simulink model "MCUSoftware"  (R2017b)
settings: Solver=FixedStepAuto  StartTime=0.0  StopTime=inf  RelTol=1e-3
undefined symbols (not defined in the file): Down, GPTRIP1SEL, GPTRIP2SEL, TZ1, TZ2, Up
libraries: c2802xlib x7, c2807xlib x2, c280xlib x1
settings Model: ExtModeTrigDuration=8  Creator=Joergen  LastModifiedBy=Joergen
settings OptimizationCC: DefaultUnderspecifiedDataType=single  PassReuseOutputArgsAs=Individual arguments  MaxStackSize=512
settings DebuggingCC: ParameterTunabilityLossMsg=error
settings HardwareCC: ProdBitPerChar=16  ProdBitPerInt=16  ProdBitPerPointer=32  ProdBitPerSizeT=32  ProdBitPerPtrDiffT=32  ProdLargestAtomicInteger=Integer  ProdLargestAtomicFloat=None  ProdWordSize=16  ProdLongLongMode=on  ProdHWDeviceType=Texas Instruments->C2000
settings SFSimCC: MATLABDynamicMemAlloc=off
settings RTWCC: SystemTargetFile=ert.tlc  HardwareBoard=TI Piccolo F2807x  TLCOptions=-aInlineSetEventsForThisBaseRateFcn=TLC_FALSE -aSuppressMultiTaskScheduler=TLC_FALSE -aRateBasedStepFcn=1  TemplateMakefile=ert_default_tmf  GenerateReport=on  Toolchain=Texas Instruments Code Composer Studio (C2000)  BuildConfiguration=Specify  IncludeHyperlinkInReport=on  LaunchReport=on  GenerateTraceInfo=on  GenerateTraceReport=on  GenerateTraceReportSl=on  GenerateTraceReportSf=on  GenerateTraceReportEml=on
settings CodeAppCC: ForceParamTrailComments=on  IgnoreCustomStorageClasses=off  OperatorAnnotations=on  SimulinkDataObjDesc=on  SFDataObjDesc=on  InsertBlockDesc=on
settings ERTTargetCC: CodeReplacementLibrary=TI C28x  SupportContinuousTime=on

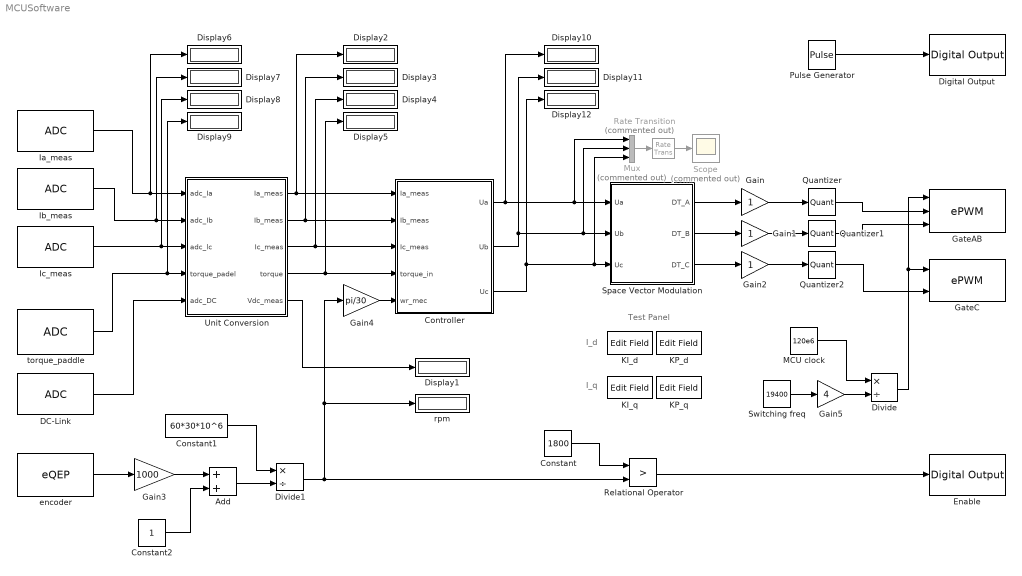
== system MCUSoftware ==
  note: I_d
  note: I_q
  note: Test Panel
  Add : Sum
  Constant : Constant  Value=1800
  Constant1 : Constant  Value=60*30*10^6
  Constant2 : Constant
  "Controller " : Subsystem
  DC-Link : c2802xlib/ADC  ADCModule=D  samplingMode=Single sample mode  ADCResolution=12-bit (Single-ended input)  useSOC1=SOC1  useSOC2=SOC0_SOC1  SOCAcquisitionWindow=12  SOCTriggerSource=ePWM1_ADCSOCA  SOCInterruptTrigger=No ADCINT  Ts=0.00001  dType=uint16  postInterrupt=off  interruptSel=ADCINT1  ADCINTContinuous=on  endma=off  chdma=1  blkParamProc=C2000_Type4  conv1=ADCINA0  conv2=ADCINA0 and ADCINB0  conv1_Type4=ADCIN1  conv2_Type4=ADCIN0 and ADCIN1
      settings: SourceProductName=Embedded Coder Support Package for Texas Instruments C2000 Processors
  Digital Output : c2807xlib/Digital Output  GPIO_Number=GPIO24~GPIO31  GPIO_Bit0=off  GPIO_BIT0_Toggle=off  GPIO_Bit1=off  GPIO_BIT1_Toggle=off  GPIO_Bit2=off  GPIO_BIT2_Toggle=off  GPIO_Bit3=off  GPIO_BIT3_Toggle=off  GPIO_Bit4=off  GPIO_BIT4_Toggle=off  GPIO_Bit5=off  GPIO_BIT5_Toggle=off  GPIO_Bit6=off  GPIO_BIT6_Toggle=on  GPIO_Bit7=on  GPIO_BIT7_Toggle=off
      settings: SourceProductName=Embedded Coder Support Package for Texas Instruments C2000 Processors  SourceProductBaseCode=TIC2000
  Display{1..12} (12 alike) : Display
  Divide : Product  Inputs=*/
  Divide1 : Product  Inputs=*/
  Enable : c2807xlib/Digital Output  GPIO_Number=GPIO8~GPIO15  GPIO_Bit0=off  GPIO_BIT0_Toggle=off  GPIO_Bit1=off  GPIO_BIT1_Toggle=off  GPIO_Bit2=off  GPIO_BIT2_Toggle=off  GPIO_Bit3=off  GPIO_BIT3_Toggle=off  GPIO_Bit4=off  GPIO_BIT4_Toggle=off  GPIO_Bit5=on  GPIO_BIT5_Toggle=off  GPIO_Bit6=off  GPIO_BIT6_Toggle=on  GPIO_Bit7=off  GPIO_BIT7_Toggle=off
      settings: SourceProductName=Embedded Coder Support Package for Texas Instruments C2000 Processors  SourceProductBaseCode=TIC2000
  Gain : Gain
  Gain1 : Gain
  Gain2 : Gain
  Gain3 : Gain  Gain=1000
  Gain4 : Gain  Gain=pi/30
  Gain5 : Gain  Gain=4
  "GateAB " : c2802xlib/ePWM  useModule=ePWM1  ePWMxLINKTBPRD=Not Linked  periodUnits=Clock cycles  timerSource=Input port  timerPeriod_clk=64000  timerPeriod_sec=0.0001  tbshadow=Counter equals to zero  countingMode=Up-Down  phaseActiveEnable=Disable  phaseDirection=Count down after sync  phaseActive=0  synchronizationEnable=off  dcaevt1Sync=off  dcbevt1Sync=off  synchronizationOption=Disable  clockPrescale=1  HSclockPrescale=1  enswap=off  ePWMxAStatus=on  ePWMxAactionLogic1=Set  ePWMxAactionLogic2=Clear  ePWMxAactionLogic3=Clear  ePWMxAactionLogic4=Set  ePWMxAactionLogic5=Do nothing  ePWMxAactionLogic6=Do nothing  ePWMxALoadMode=Load on counter equals to zero (CTR=Zero)  ePWMxACSFenable=off  ePWMxACSFvalue=Forcing disable  ePWMxASFreload=Zero  ePWMxBStatus=on  ePWMxBactionLogic1=Set  ePWMxBactionLogic2=Clear  ePWMxBactionLogic3=Do nothing  ePWMxBactionLogic4=Do nothing  ePWMxBactionLogic5=Clear  ePWMxBactionLogic6=Set  ePWMxBLoadMode=Load on counter equals to zero (CTR=Zero)  ePWMxBCSFenable=off  ePWMxBCSFvalue=Forcing disable  ePWMxBSFreload=Zero  ePWNxBOutWay=off  ePWMxLINKCMPA=Not Linked  CMPAUnits=Percentages  CMPASource=Input port  CMPAValue_per=50  CMPAValue_clk=0  enCMPAshadow=Counter equals to zero  ePWMxLINKCMPB=Not Linked  CMPBUnits=Percentages  CMPBSource=Input port  CMPBValue_per=50  CMPBValue_clk=0  enCMPBshadow=Counter equals to zero  ePWMxLINKCMPC=Not Linked  CMPCUnits=Clock cycles  CMPCSource=Specify via dialog  CMPCValue_per=50  CMPCValue_clk=32000  enCMPCshadow=Counter equals to zero  ePWMxLINKCMPD=Not Linked  CMPDUnits=Clock cycles  CMPDSource=Specify via dialog  CMPDValue_per=50  CMPDValue_clk=32000  enCMPDshadow=Counter equals to zero  enableDBePWMxA=off  enableDBePWMxB=off  enhalfcycle=off  DBpolarity=Active high (AH)  DBedgeDelay=Positive  DBSource_ePWMxA=ePWMxA  DBSource_ePWMxB=ePWMxA  DBperiodSource=Specify via dialog  REDperiod=0  FEDperiod=0  adcstartModuleA=on  adcrequestEventA=First event  adcstartEventA=Digital Compare Module A Event 1 start of conversion (DCAEVT1.soc)  adcstartEventA_type2=Counter equals to period (CTR=PRD)  adcstartModuleB=off  adcrequestEventB=First event  adcstartEventB=Counter equals to zero (CTR=Zero)  adcstartEventB_type2=Counter equals to zero (CTR=Zero)  intEn=off  intPrd=First event  intSel=Counter equals to zero (CTR=Zero)  intSel_type2=Counter equals to zero (CTR=Zero)  hrpe=off  enHRPWM=off  HRPWM_LoadMode=Counter equals to period (CTR=PRD)  HRPWM_CTLMode=Duty or Period control mode  HRPWM_EDGMode=Both edge  hrpeb=off  enHRPWMB=off  HRPWM_LoadModeB=Counter equals to zero (CTR=ZERO)  HRPWM_CTLModeB=Duty or Period control mode  HRPWM_EDGModeB=Both edge  enSFO=on  enautoconv=on  chopperEnable=off  chopperFrequency=1  chopperFirstwidth=1  chopperDuty=12.5%  tripZonesource=Specify via dialog  tzselOSHT1=off  tzselOSHT2=off  tzselOSHT3=off  tzselOSHDCAEV1=off  tzselOSHDCBEV1=off  tzselCBC1=off  tzselCBC2=off  tzselCBC3=off  tzselCBCDCAEV2=off  tzselCBCDCBEV2=off  tzselOSHT4=off  tzselOSHT5=off  tzselOSHT6=off  tzselCBC4=off  tzselCBC5=off  tzselCBC6=off  enTzOstIntr=off  enTzCbcIntr=off  enTzDCAEVT1Intr=off  enTzDCAEVT2Intr=off  enTzDCBEVT1Intr=off  enTzDCBEVT2Intr=off  ePWMxAforced=No action  ePWMxBforced=No action  DCAEVT1forced=No action  DCBEVT1forced=No action  DCAEVT2forced=No action  DCBEVT2forced=No action  dcah=Trip Zone 1 input (TZ1)  dcal=Trip Zone 2 input (TZ2)  dcbh=Trip Zone 1 input (TZ1)  dcbl=Trip Zone 2 input (TZ2)  dcah_type2=GPTRIP1SEL/(TZ1)  dcal_type2=GPTRIP2SEL/(TZ2)  dcbh_type2=GPTRIP1SEL/(TZ1)  dcbl_type2=GPTRIP2SEL/(TZ2)  gendcaevt1=Event disabled  gendcaevt2=Event disabled  gendcbevt1=Event disabled  gendcbevt2=Event disabled  dcaevt1src=DCAEVT1 with sync  dcaevt2src=DCAEVT2 with sync  dcbevt1src=DCBEVT1 with sync  dcbevt2src=DCBEVT2 with sync  pulsesel=Counter equals to zero (CTR=Zero)  blankinv=off  blankoffset=0  blankwidth=0  evsrcsel=Filtered version of DCAEVT1 (DCAEVT1FILT)  encape=off  PwmType=C2000_Type4
      settings: SourceProductName=Embedded Coder Support Package for Texas Instruments C2000 Processors
  GateC : c2802xlib/ePWM  useModule=ePWM2  ePWMxLINKTBPRD=Not Linked  periodUnits=Clock cycles  timerSource=Input port  timerPeriod_clk=64000  timerPeriod_sec=0.0001  tbshadow=Counter equals to zero  countingMode=Up-Down  phaseActiveEnable=Disable  phaseDirection=Count down after sync  phaseActive=0  synchronizationEnable=off  dcaevt1Sync=off  dcbevt1Sync=off  synchronizationOption=Disable  clockPrescale=1  HSclockPrescale=1  enswap=off  ePWMxAStatus=on  ePWMxAactionLogic1=Set  ePWMxAactionLogic2=Clear  ePWMxAactionLogic3=Clear  ePWMxAactionLogic4=Set  ePWMxAactionLogic5=Do nothing  ePWMxAactionLogic6=Do nothing  ePWMxALoadMode=Load on counter equals to zero (CTR=Zero)  ePWMxACSFenable=off  ePWMxACSFvalue=Forcing disable  ePWMxASFreload=Zero  ePWMxBStatus=off  ePWMxBactionLogic1=Set  ePWMxBactionLogic2=Clear  ePWMxBactionLogic3=Do nothing  ePWMxBactionLogic4=Do nothing  ePWMxBactionLogic5=Clear  ePWMxBactionLogic6=Set  ePWMxBLoadMode=Load on counter equals to zero (CTR=Zero)  ePWMxBCSFenable=off  ePWMxBCSFvalue=Forcing disable  ePWMxBSFreload=Zero  ePWNxBOutWay=off  ePWMxLINKCMPA=Not Linked  CMPAUnits=Percentages  CMPASource=Input port  CMPAValue_per=50  CMPAValue_clk=0  enCMPAshadow=Counter equals to zero  ePWMxLINKCMPB=Not Linked  CMPBUnits=Clock cycles  CMPBSource=Specify via dialog  CMPBValue_per=50  CMPBValue_clk=32000  enCMPBshadow=Counter equals to zero  ePWMxLINKCMPC=Not Linked  CMPCUnits=Clock cycles  CMPCSource=Specify via dialog  CMPCValue_per=50  CMPCValue_clk=32000  enCMPCshadow=Counter equals to zero  ePWMxLINKCMPD=Not Linked  CMPDUnits=Clock cycles  CMPDSource=Specify via dialog  CMPDValue_per=50  CMPDValue_clk=32000  enCMPDshadow=Counter equals to zero  enableDBePWMxA=off  enableDBePWMxB=off  enhalfcycle=off  DBpolarity=Active high (AH)  DBedgeDelay=Positive  DBSource_ePWMxA=ePWMxA  DBSource_ePWMxB=ePWMxA  DBperiodSource=Specify via dialog  REDperiod=0  FEDperiod=0  adcstartModuleA=off  adcrequestEventA=First event  adcstartEventA=Digital Compare Module A Event 1 start of conversion (DCAEVT1.soc)  adcstartEventA_type2=Digital Compare Module A Event 1 start of conversion (DCAEVT1.soc)  adcstartModuleB=off  adcrequestEventB=First event  adcstartEventB=Counter equals to zero (CTR=Zero)  adcstartEventB_type2=Counter equals to zero (CTR=Zero)  intEn=off  intPrd=First event  intSel=Counter equals to zero (CTR=Zero)  intSel_type2=Counter equals to zero (CTR=Zero)  hrpe=off  enHRPWM=off  HRPWM_LoadMode=Counter equals to period (CTR=PRD)  HRPWM_CTLMode=Duty or Period control mode  HRPWM_EDGMode=Both edge  hrpeb=off  enHRPWMB=off  HRPWM_LoadModeB=Counter equals to zero (CTR=ZERO)  HRPWM_CTLModeB=Duty or Period control mode  HRPWM_EDGModeB=Both edge  enSFO=on  enautoconv=on  chopperEnable=off  chopperFrequency=1  chopperFirstwidth=1  chopperDuty=12.5%  tripZonesource=Specify via dialog  tzselOSHT1=off  tzselOSHT2=off  tzselOSHT3=off  tzselOSHDCAEV1=off  tzselOSHDCBEV1=off  tzselCBC1=off  tzselCBC2=off  tzselCBC3=off  tzselCBCDCAEV2=off  tzselCBCDCBEV2=off  tzselOSHT4=off  tzselOSHT5=off  tzselOSHT6=off  tzselCBC4=off  tzselCBC5=off  tzselCBC6=off  enTzOstIntr=off  enTzCbcIntr=off  enTzDCAEVT1Intr=off  enTzDCAEVT2Intr=off  enTzDCBEVT1Intr=off  enTzDCBEVT2Intr=off  ePWMxAforced=No action  ePWMxBforced=No action  DCAEVT1forced=No action  DCBEVT1forced=No action  DCAEVT2forced=No action  DCBEVT2forced=No action  dcah=Trip Zone 1 input (TZ1)  dcal=Trip Zone 2 input (TZ2)  dcbh=Trip Zone 1 input (TZ1)  dcbl=Trip Zone 2 input (TZ2)  dcah_type2=GPTRIP1SEL/(TZ1)  dcal_type2=GPTRIP2SEL/(TZ2)  dcbh_type2=GPTRIP1SEL/(TZ1)  dcbl_type2=GPTRIP2SEL/(TZ2)  gendcaevt1=Event disabled  gendcaevt2=Event disabled  gendcbevt1=Event disabled  gendcbevt2=Event disabled  dcaevt1src=DCAEVT1 with sync  dcaevt2src=DCAEVT2 with sync  dcbevt1src=DCBEVT1 with sync  dcbevt2src=DCBEVT2 with sync  pulsesel=Counter equals to zero (CTR=Zero)  blankinv=off  blankoffset=0  blankwidth=0  evsrcsel=Filtered version of DCAEVT1 (DCAEVT1FILT)  encape=off  PwmType=C2000_Type4
      settings: SourceProductName=Embedded Coder Support Package for Texas Instruments C2000 Processors
  Ia_meas : c2802xlib/ADC  ADCModule=A  samplingMode=Single sample mode  ADCResolution=12-bit (Single-ended input)  useSOC1=SOC0  useSOC2=SOC0_SOC1  SOCAcquisitionWindow=12  SOCTriggerSource=ePWM1_ADCSOCA  SOCInterruptTrigger=No ADCINT  Ts=0.00001  dType=uint16  postInterrupt=off  interruptSel=ADCINT1  ADCINTContinuous=on  endma=off  chdma=1  blkParamProc=C2000_Type4  conv1=ADCINA0  conv2=ADCINA0 and ADCINB0  conv1_Type4=ADCIN0  conv2_Type4=ADCIN0 and ADCIN1
      settings: SourceProductName=Embedded Coder Support Package for Texas Instruments C2000 Processors
  "Ib_meas " : c2802xlib/ADC  ADCModule=B  samplingMode=Single sample mode  ADCResolution=12-bit (Single-ended input)  useSOC1=SOC0  useSOC2=SOC0_SOC1  SOCAcquisitionWindow=12  SOCTriggerSource=ePWM1_ADCSOCA  SOCInterruptTrigger=ADCINT1  Ts=0.00001  dType=uint16  postInterrupt=off  interruptSel=ADCINT1  ADCINTContinuous=on  endma=off  chdma=1  blkParamProc=C2000_Type4  conv1=ADCINA0  conv2=ADCINA0 and ADCINB0  conv1_Type4=ADCIN0  conv2_Type4=ADCIN0 and ADCIN1
      settings: SourceProductName=Embedded Coder Support Package for Texas Instruments C2000 Processors
  "Ic_meas " : c2802xlib/ADC  ADCModule=D  samplingMode=Single sample mode  ADCResolution=12-bit (Single-ended input)  useSOC1=SOC0  useSOC2=SOC0_SOC1  SOCAcquisitionWindow=12  SOCTriggerSource=ePWM1_ADCSOCA  SOCInterruptTrigger=ADCINT1  Ts=0.00001  dType=uint16  postInterrupt=off  interruptSel=ADCINT1  ADCINTContinuous=on  endma=off  chdma=1  blkParamProc=C2000_Type4  conv1=ADCINA0  conv2=ADCINA0 and ADCINB0  conv1_Type4=ADCIN0  conv2_Type4=ADCIN0 and ADCIN1
      settings: SourceProductName=Embedded Coder Support Package for Texas Instruments C2000 Processors
  KI_d : EditField  WebBlockId=101  ModelName=MCUSoftware  LabelPosition=Hide  ShowInitialText=off  Alignment=Center
  KI_q : EditField  WebBlockId=102  ModelName=MCUSoftware  LabelPosition=Hide  ShowInitialText=off  Alignment=Center
  KP_d : EditField  WebBlockId=103  ModelName=MCUSoftware  LabelPosition=Hide  ShowInitialText=off  Alignment=Center
  KP_q : EditField  WebBlockId=104  ModelName=MCUSoftware  LabelPosition=Hide  ShowInitialText=off  Alignment=Center
  MCU clock : Constant  Value=120e6
  Mux : Mux  Commented=on  Inputs=3
  Pulse Generator : DiscretePulseGenerator  PulseType=Time based  Period=0.5  PulseWidth=90
  Quantizer : Quantizer  QuantizationInterval=0.001
  Quantizer1 : Quantizer  QuantizationInterval=0.001
  Quantizer2 : Quantizer  QuantizationInterval=0.001
  Rate Transition : RateTransition  Commented=on
  Relational Operator : RelationalOperator  Operator=>  RndMeth=Simplest
  Scope : Scope  Commented=on
  Space Vector Modulation : Subsystem
  Switching freq : Constant  Value=19400
  Unit Conversion : Subsystem
  encoder : c280xlib/eQEP  useModule=eQEP1  pcInputmode=Quadrature-count  externalClockrate=2x resolution: Count the rising/falling edge  swapPolarityselection=Clockwise  qdfOutputport=off  qapPolarityselection=off  qbpPolarityselection=off  qipPolarityselection=off  qspPolarityselection=off  igatePolarityselection=off  sampleTime=0.00001  pcOutputport=off  pcMaximumvalue=4294967295  indexInitializationcheck=off  indexInitializationevent=Rising edge  strobeInitializationcheck=off  strobeInitializationevent=Rising edge  softwareInitializationcheck=off  softwareInitializationsource=Set to init value at start up  softwareInitializationmode=on  pcInitialvalue=2147483648  pcResetmode=Reset on an index event  ieloutputport=off  indexEventlatch=Rising edge  seloutputport=off  strobeEventlatch=Rising edge  pcefOutputport=off  enableEqepcapture=on  qctmrOutputport=off  qcprdOutputport=on  captureTimerprescaler=128  upEventprescaler=128  overflowErrorflag=off  directionErrorflag=off  captureTimerposition=On position counter read  unitTimerperiod=100000000  captureTimerlatch=off  capturePeriodlatch=off  positionCounterlatch=off  soenPolarityselection=off  spselPolarityselection=Index pin is used for sync output  compareValuesource=Specify via dialog  shadowMode=Load on QPOSCNT=0  compareValue=4294967295  syncOutputwidth=1  polaritySyncoutput=Active high  watchdogEnable=off  watchdogTimer=65535  outport1Datatype=auto  outport2Datatype=auto  outport3Datatype=auto  outport4Datatype=auto  outport5Datatype=auto  outport6Datatype=auto  outport7Datatype=auto  outport8Datatype=auto  outport9Datatype=auto  outport10Datatype=auto  outport11Datatype=auto  outport12Datatype=auto  eqepinterrupt_pce=off  eqepinterrupt_qpe=off  eqepinterrupt_qdc=off  eqepinterrupt_wto=off  eqepinterrupt_pcu=off  eqepinterrupt_pco=off  eqepinterrupt_pcr=off  eqepinterrupt_pcm=off  eqepinterrupt_sel=off  eqepinterrupt_iel=off  eqepinterrupt_uto=off  pheOutputport=off  watchdogOutputport=off  outport13Datatype=auto  outport14Datatype=auto
      settings: SourceProductName=Embedded Coder Support Package for Texas Instruments C2000 Processors  SourceProductBaseCode=TIC2000
  rpm : Display
  torque_paddle : c2802xlib/ADC  ADCModule=B  samplingMode=Single sample mode  ADCResolution=12-bit (Single-ended input)  useSOC1=SOC1  useSOC2=SOC0_SOC1  SOCAcquisitionWindow=12  SOCTriggerSource=ePWM1_ADCSOCA  SOCInterruptTrigger=No ADCINT  Ts=0.00001  dType=uint16  postInterrupt=off  interruptSel=ADCINT1  ADCINTContinuous=on  endma=off  chdma=1  blkParamProc=C2000_Type4  conv1=ADCINA0  conv2=ADCINA0 and ADCINB0  conv1_Type4=ADCIN1  conv2_Type4=ADCIN0 and ADCIN1
      settings: SourceProductName=Embedded Coder Support Package for Texas Instruments C2000 Processors
  wires:
  torque_paddle/1 -> Unit Conversion/4(torque_padel), Display9/1
  Unit Conversion/3(Ic_meas) -> Display4/1, "Controller "/3(Ic_meas)
  "Ic_meas "/1 -> Unit Conversion/3(adc_lc), Display8/1
  Unit Conversion/2(Ib_meas) -> Display3/1, "Controller "/2(Ib_meas)
  "Ib_meas "/1 -> Unit Conversion/2(adc_Ib), Display7/1
  Relational Operator/1 -> Enable/1
  Gain2/1 -> Quantizer2/1
  Divide/1 -> "GateAB "/1, GateC/1
  Gain1/1 -> Quantizer1/1
  "Controller "/3(Uc) -> Space Vector Modulation/3(Uc), Mux/3, Display12/1
  Unit Conversion/4(torque) -> Display5/1, "Controller "/4(torque_in)
  Mux/1 -> Rate Transition/1
  Space Vector Modulation/3(DT_C) -> Gain2/1
  Space Vector Modulation/1(DT_A) -> Gain/1
  "Controller "/2(Ub) -> Mux/2, Space Vector Modulation/2(Ub), Display11/1
  Space Vector Modulation/2(DT_B) -> Gain1/1
  Ia_meas/1 -> Display6/1, Unit Conversion/1(adc_Ia)
  Gain/1 -> Quantizer/1
  DC-Link/1 -> Unit Conversion/5(adc_DC)
  Unit Conversion/5(Vdc_meas) -> Display1/1
  Quantizer/1 -> "GateAB "/2
  Quantizer1/1 -> "GateAB "/3
  Quantizer2/1 -> GateC/2
  Pulse Generator/1 -> Digital Output/1
  Unit Conversion/1(Ia_meas) -> "Controller "/1(Ia_meas), Display2/1
  MCU clock/1 -> Divide/1
  Switching freq/1 -> Gain5/1
  Rate Transition/1 -> Scope/1
  "Controller "/1(Ua) -> Space Vector Modulation/1(Ua), Mux/1, Display10/1
  Divide1/1 -> Relational Operator/2, Gain4/1, rpm/1
  Gain3/1 -> Add/1
  Constant1/1 -> Divide1/1
  Gain4/1 -> "Controller "/5(wr_mec)
  Gain5/1 -> Divide/2
  Constant/1 -> Relational Operator/1
  Add/1 -> Divide1/2
  encoder/1 -> Gain3/1
  Constant2/1 -> Add/2

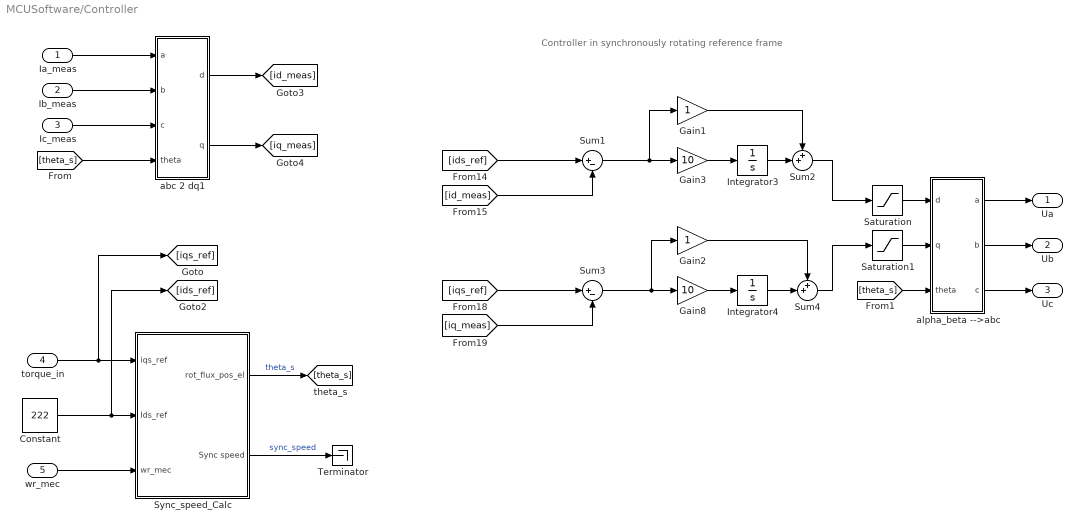
== system MCUSoftware/Controller  ==
  note: Controller in synchronously rotating reference frame
  Ia_meas : Inport
  Ib_meas : Inport  Port=2
  Ic_meas : Inport  Port=3
  torque_in : Inport  Port=4
  wr_mec : Inport  Port=5
  " alpha_beta -->abc" : Subsystem
  Constant : Constant  Value=222
  Gain1 : Gain  SaturateOnIntegerOverflow=on  OutDataTypeStr=Inherit: Same as input  ParamDataTypeStr=Inherit: Same as input
  Gain2 : Gain  SaturateOnIntegerOverflow=on  OutDataTypeStr=Inherit: Same as input  ParamDataTypeStr=Inherit: Same as input
  Gain3 : Gain  Gain=10  SaturateOnIntegerOverflow=on  OutDataTypeStr=Inherit: Same as input  ParamDataTypeStr=Inherit: Same as input
  Gain8 : Gain  Gain=10  SaturateOnIntegerOverflow=on  OutDataTypeStr=Inherit: Same as input  ParamDataTypeStr=Inherit: Same as input
  Integrator3 : Integrator
  Integrator4 : Integrator
  Saturation : Saturate  UpperLimit=34  LowerLimit=-34
  Saturation1 : Saturate  UpperLimit=34  LowerLimit=-34
  Sum1 : Sum  Inputs=|+-  SaturateOnIntegerOverflow=on  InputSameDT=on  OutDataTypeStr=Inherit: Same as first input
  Sum2 : Sum  Inputs=++|  SaturateOnIntegerOverflow=on  InputSameDT=on  OutDataTypeStr=Inherit: Same as first input
  Sum3 : Sum  Inputs=|+-  SaturateOnIntegerOverflow=on  InputSameDT=on  OutDataTypeStr=Inherit: Same as first input
  Sum4 : Sum  Inputs=++|  SaturateOnIntegerOverflow=on  InputSameDT=on  OutDataTypeStr=Inherit: Same as first input
  Sync_speed_Calc : Subsystem
  Terminator : Terminator
  abc 2 dq1 : Subsystem
  Ua : Outport
  Ub : Outport  Port=2
  Uc : Outport  Port=3
  wires:
  Ia_meas/1 -> abc 2 dq1/1(a)
  Ic_meas/1 -> abc 2 dq1/3(c)
  torque_in/1 -> [iqs_ref], Sync_speed_Calc/1(iqs_ref)
  Constant/1 -> [ids_ref], Sync_speed_Calc/2(Ids_ref)
  wr_mec/1 -> Sync_speed_Calc/3(wr_mec)
  Sync_speed_Calc/1(rot_flux_pos_el) -> [theta_s]  "theta_s"
  [theta_s] -> abc 2 dq1/4(theta)
  Integrator4/1 -> Sum4/2
  Integrator3/1 -> Sum2/2
  [iq_meas] -> Sum3/2
  [iqs_ref] -> Sum3/1
  Gain8/1 -> Integrator4/1
  Gain3/1 -> Integrator3/1
  Sum4/1 -> Saturation1/1
  abc 2 dq1/1(d) -> [id_meas]
  abc 2 dq1/2(q) -> [iq_meas]
  [theta_s] -> " alpha_beta -->abc"/3(theta)
  Sum2/1 -> Saturation/1
  Ib_meas/1 -> abc 2 dq1/2(b)
  Sum1/1 -> Gain1/1, Gain3/1
  [id_meas] -> Sum1/2
  [ids_ref] -> Sum1/1
  " alpha_beta -->abc"/1(a) -> Ua/1
  " alpha_beta -->abc"/2(b) -> Ub/1
  Gain1/1 -> Sum2/1
  Gain2/1 -> Sum4/1
  Sum3/1 -> Gain8/1, Gain2/1
  " alpha_beta -->abc"/3(c) -> Uc/1
  Saturation/1 -> " alpha_beta -->abc"/1(d)
  Saturation1/1 -> " alpha_beta -->abc"/2(q)
  Sync_speed_Calc/2(Sync speed) -> Terminator/1  "sync_speed"

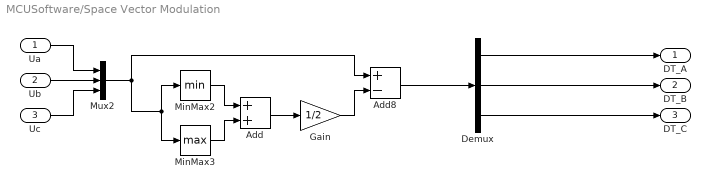
== system MCUSoftware/Space Vector Modulation ==
  Ua : Inport
  Ub : Inport  Port=2
  Uc : Inport  Port=3
  Add : Sum
  Add8 : Sum  Inputs=+-
  Demux : Demux  Outputs=3
  Gain : Gain  Gain=1/2
  MinMax2 : MinMax
  MinMax3 : MinMax  Function=max
  Mux2 : Mux  Inputs=3
  DT_A : Outport
  DT_B : Outport  Port=2
  DT_C : Outport  Port=3
  wires:
  MinMax2/1 -> Add/1
  Add/1 -> Gain/1
  Gain/1 -> Add8/2
  Uc/1 -> Mux2/3
  Ub/1 -> Mux2/2
  Demux/3 -> DT_C/1
  Ua/1 -> Mux2/1
  Demux/2 -> DT_B/1
  Demux/1 -> DT_A/1
  MinMax3/1 -> Add/2
  Mux2/1 -> MinMax2/1, MinMax3/1, Add8/1
  Add8/1 -> Demux/1

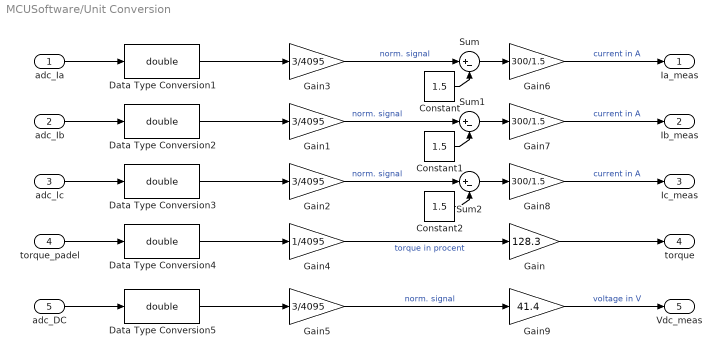
== system MCUSoftware/Unit Conversion ==
  adc_Ia : Inport
  adc_Ib : Inport  Port=2
  adc_lc : Inport  Port=3
  torque_padel : Inport  Port=4
  adc_DC : Inport  Port=5
  Constant : Constant  Value=1.5
  Constant1 : Constant  Value=1.5
  Constant2 : Constant  Value=1.5
  Data Type Conversion{1..5} (5 alike) : DataTypeConversion  OutDataTypeStr=double
  Gain : Gain  Gain=128.3
  Gain{1..3,5} (4 alike) : Gain  Gain=3/4095
  Gain4 : Gain  Gain=1/4095
  Gain6 : Gain  Gain=300/1.5
  Gain7 : Gain  Gain=300/1.5
  Gain8 : Gain  Gain=300/1.5
  Gain9 : Gain  Gain=41.4
  Sum : Sum  Inputs=|+-
  Sum1 : Sum  Inputs=|+-
  Sum2 : Sum  Inputs=|+-
  Ia_meas : Outport
  Ib_meas : Outport  Port=2
  Ic_meas : Outport  Port=3
  torque : Outport  Port=4
  Vdc_meas : Outport  Port=5
  wires:
  Gain4/1 -> Gain/1  "torque in procent"
  adc_Ib/1 -> Data Type Conversion2/1
  adc_lc/1 -> Data Type Conversion3/1
  adc_Ia/1 -> Data Type Conversion1/1
  torque_padel/1 -> Data Type Conversion4/1
  adc_DC/1 -> Data Type Conversion5/1
  Gain5/1 -> Gain9/1  "norm. signal"
  Data Type Conversion1/1 -> Gain3/1
  Data Type Conversion2/1 -> Gain1/1
  Data Type Conversion3/1 -> Gain2/1
  Data Type Conversion4/1 -> Gain4/1
  Data Type Conversion5/1 -> Gain5/1
  Gain6/1 -> Ia_meas/1  "current in A"
  Gain7/1 -> Ib_meas/1  "current in A"
  Gain8/1 -> Ic_meas/1  "current in A"
  Gain9/1 -> Vdc_meas/1  "voltage in V"
  Constant/1 -> Sum/2
  Gain3/1 -> Sum/1  "norm. signal"
  Sum/1 -> Gain6/1
  Constant1/1 -> Sum1/2
  Constant2/1 -> Sum2/2
  Gain2/1 -> Sum2/1  "norm. signal"
  Sum2/1 -> Gain8/1
  Gain1/1 -> Sum1/1  "norm. signal"
  Sum1/1 -> Gain7/1
  Gain/1 -> torque/1

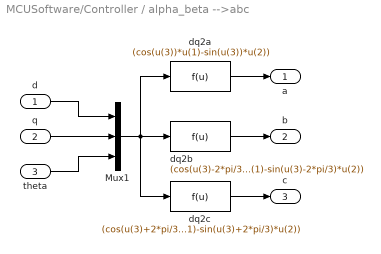
== system MCUSoftware/Controller / alpha_beta -->abc ==
  d : Inport
  q : Inport  Port=2
  theta : Inport  Port=3
  Mux1 : Mux  Inputs=3
  dq2a : Fcn  Expr=(cos(u(3))*u(1)-sin(u(3))*u(2))
  dq2b : Fcn  Expr=(cos(u(3)-2*pi/3)*u(1)-sin(u(3)-2*pi/3)*u(2))
  dq2c : Fcn  Expr=(cos(u(3)+2*pi/3)*u(1)-sin(u(3)+2*pi/3)*u(2))
  a : Outport
  b : Outport  Port=2
  c : Outport  Port=3
  wires:
  dq2b/1 -> b/1
  dq2a/1 -> a/1
  Mux1/1 -> dq2c/1, dq2b/1, dq2a/1
  d/1 -> Mux1/1
  theta/1 -> Mux1/3
  q/1 -> Mux1/2
  dq2c/1 -> c/1

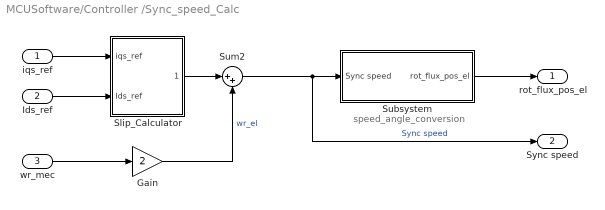
== system MCUSoftware/Controller /Sync_speed_Calc ==
  note: speed_angle_conversion
  iqs_ref : Inport
  Ids_ref : Inport  Port=2
  wr_mec : Inport  Port=3
  Gain : Gain  Gain=2
  Slip_Calculator : Subsystem
  Subsystem : Subsystem
  Sum2 : Sum  Inputs=|++
  rot_flux_pos_el : Outport
  Sync speed : Outport  Port=2
  wires:
  Gain/1 -> Sum2/2  "wr_el"
  Slip_Calculator/1(slip speed) -> Sum2/1
  Subsystem/1(rot_flux_pos_el) -> rot_flux_pos_el/1
  wr_mec/1 -> Gain/1
  Ids_ref/1 -> Slip_Calculator/2(Ids_ref)
  iqs_ref/1 -> Slip_Calculator/1(iqs_ref)
  Sum2/1 -> Sync speed/1, Subsystem/1(Sync speed)  "Sync speed"

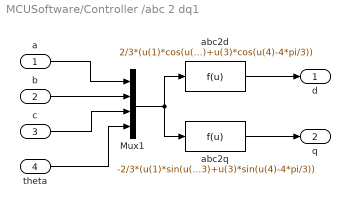
== system MCUSoftware/Controller /abc 2 dq1 ==
  a : Inport
  b : Inport  Port=2
  c : Inport  Port=3
  theta : Inport  Port=4
  Mux1 : Mux
  abc2d : Fcn  Expr=2/3*(u(1)*cos(u(4))+u(2)*cos(u(4)-2*pi/3)+u(3)*cos(u(4)-4*pi/3))
  abc2q : Fcn  Expr=-2/3*(u(1)*sin(u(4))+u(2)*sin(u(4)-2*pi/3)+u(3)*sin(u(4)-4*pi/3))
  d : Outport
  q : Outport  Port=2
  wires:
  Mux1/1 -> abc2q/1, abc2d/1
  abc2q/1 -> q/1
  a/1 -> Mux1/1
  b/1 -> Mux1/2
  c/1 -> Mux1/3
  theta/1 -> Mux1/4
  abc2d/1 -> d/1

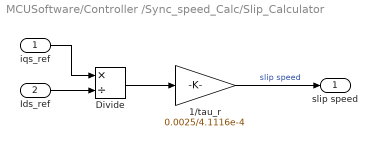
== system MCUSoftware/Controller /Sync_speed_Calc/Slip_Calculator ==
  iqs_ref : Inport
  Ids_ref : Inport  Port=2
  1/tau_r : Gain  Gain=0.0025/4.1116e-4
  Divide : Product  Inputs=*/
  slip speed : Outport
  wires:
  Ids_ref/1 -> Divide/2
  iqs_ref/1 -> Divide/1
  Divide/1 -> 1/tau_r/1
  1/tau_r/1 -> slip speed/1  "slip speed"

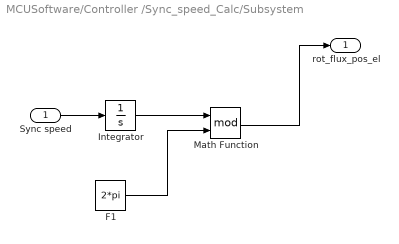
== system MCUSoftware/Controller /Sync_speed_Calc/Subsystem ==
  Sync speed : Inport
  F1 : Constant  Value=2*pi
  Integrator : Integrator
  Math Function : Math  Operator=mod  SaturateOnIntegerOverflow=on
  rot_flux_pos_el : Outport
  wires:
  Integrator/1 -> Math Function/1
  Math Function/1 -> rot_flux_pos_el/1
  F1/1 -> Math Function/2
  Sync speed/1 -> Integrator/1
